simulink model "DAC"  (Simulink 9.3)
settings: Solver=ode3  StartTime=0.0  StopTime=5*T0  FixedStep=Te  RelTol=1e-3  EnableMultiTasking=on
InitFcn:
  | DAC_InitFcn()
StopFcn:
  | DAC_StopFcn()
values from neighbouring files (symbols this model uses):
  F0 = 50    [DAC_InitFcn.m]
  SD = 100    [DAC_InitFcn.m]
  Tau = 2*pi/Fe    (= 1.25663706144e-05)    [DAC_InitFcn.m]
  Te = 1/Fe    (= 2e-06)    [DAC_InitFcn.m]
  W = [32 16 8 4 2 1 1 1 1]'    [DAC_InitFcn.m]
libraries: dsparch4 x1
settings Model: Creator=F555267  LastModifiedBy=Fatwir SM
settings SolverCC: AutoInsertRateTranBlk=on
settings DataIOCC: LimitDataPoints=on
settings OptimizationCC: ExpressionDepthLimit=2147483647
settings DebuggingCC: SolverPrmCheckMsg=warning  StateNameClashWarn=warning
settings GRTTargetCC: GeneratePreprocessorConditionals=Disable all
settings ConfigComp: CovSFcnEnable=off

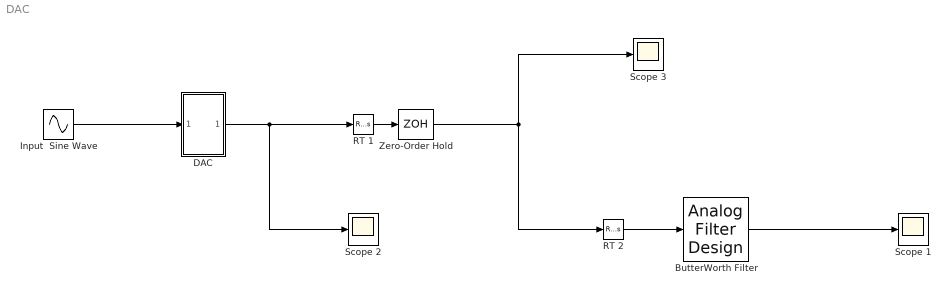
== system DAC ==
  ButterWorth Filter : dsparch4/Analog Filter Design  method=Butterworth  filttype=Lowpass  N=5  Wlo=2*pi*50  Whi=80  Rp=2  Rs=40
  DAC : Subsystem
  Input  Sine Wave : Sin  Amplitude=SD  Frequency=2*pi*F0  SampleTime=0
  RT 1 : RateTransition  OutPortSampleTimeOpt=Inherit  OutPortSampleTime=4e-06
  RT 2 : RateTransition  OutPortSampleTimeOpt=Inherit  OutPortSampleTimeMultiple=2*Tau  OutPortSampleTime=2e-06
  Scope 1 : Scope
  Scope 2 : Scope
  Scope 3 : Scope
  Zero-Order Hold : ZeroOrderHold  SampleTime=100*Te
  wires:
  RT 2/1 -> ButterWorth Filter/1
  RT 1/1 -> Zero-Order Hold/1
  Input  Sine Wave/1 -> DAC/1(In1)
  Zero-Order Hold/1 -> Scope 3/1, RT 2/1
  ButterWorth Filter/1 -> Scope 1/1
  DAC/1(Out1) -> Scope 2/1, RT 1/1

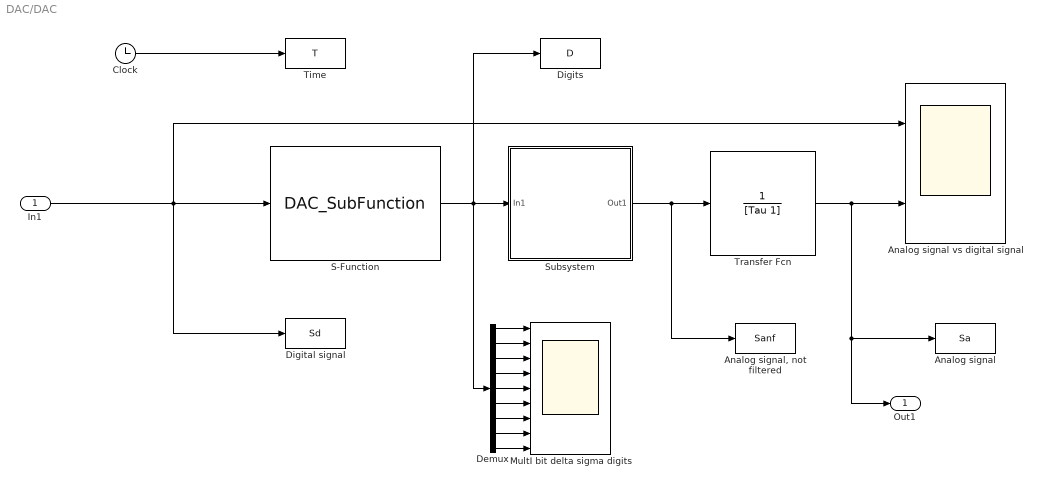
== system DAC/DAC ==
  In1 : Inport
  Analog signal : ToWorkspace  VariableName=Sa  SampleTime=-1
      settings: Save2DSignal=2-D array (concatenate along first dimension)
  Analog signal vs digital signal : Scope  NumInputPorts=2
  "Analog signal, not filtered" : ToWorkspace  VariableName=Sanf  SampleTime=-1
      settings: Save2DSignal=2-D array (concatenate along first dimension)
  Clock : Clock
  Demux : Demux  Outputs=9
  Digital signal : ToWorkspace  VariableName=Sd  SampleTime=-1
  Digits : ToWorkspace  VariableName=D  SampleTime=-1
      settings: Save2DSignal=2-D array (concatenate along first dimension)
  MultI bit delta sigma digits : Scope  NumInputPorts=9
  S-Function : S-Function  FunctionName=DAC_SubFunction  SFunctionDeploymentMode=off  EnableBusSupport=off
      mask Display: disp('Multi bit delta sigma DAC')
  Subsystem : Subsystem
      mask Display: disp('Summation')
  Time : ToWorkspace  VariableName=T  SampleTime=-1
  Transfer Fcn : TransferFcn  Numerator=1  Denominator=[Tau 1]
      mask Display: disp('Low pass filter')
  Out1 : Outport
  wires:
  Demux/8 -> MultI bit delta sigma digits/8
  Demux/6 -> MultI bit delta sigma digits/6
  Transfer Fcn/1 -> Analog signal vs digital signal/2, Analog signal/1, Out1/1
  Demux/9 -> MultI bit delta sigma digits/9
  Clock/1 -> Time/1
  Demux/2 -> MultI bit delta sigma digits/2
  Demux/1 -> MultI bit delta sigma digits/1
  Demux/7 -> MultI bit delta sigma digits/7
  S-Function/1 -> Subsystem/1(In1), Digits/1, Demux/1
  Demux/5 -> MultI bit delta sigma digits/5
  In1/1 -> S-Function/1, Digital signal/1, Analog signal vs digital signal/1
  Subsystem/1(Out1) -> "Analog signal, not filtered"/1, Transfer Fcn/1
  Demux/4 -> MultI bit delta sigma digits/4
  Demux/3 -> MultI bit delta sigma digits/3

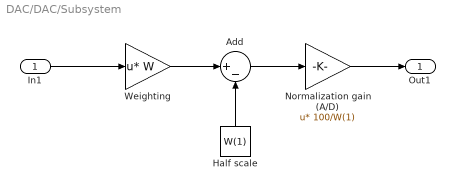
== system DAC/DAC/Subsystem ==
  In1 : Inport
  Add : Sum  Inputs=|+-
  Half scale : Constant  Value=W(1)
  Normalization gain (A/D) : Gain  Gain=100/W(1)  Multiplication=Matrix(u*K)
  Weighting : Gain  Gain=W  Multiplication=Matrix(u*K)
  Out1 : Outport
  wires:
  In1/1 -> Weighting/1
  Weighting/1 -> Add/1
  Add/1 -> Normalization gain (A/D)/1
  Half scale/1 -> Add/2
  Normalization gain (A/D)/1 -> Out1/1
